simulink model "main"  (R2023a)
settings: Solver=VariableStepAuto  StartTime=0.0  StopTime=20.0  RelTol=1e-3
values from neighbouring files (symbols this model uses):
  K_cor = -321.168335055129    (= -321.168335055)    [init_constants.m]
  K_d = -25.0617020806048    (= -25.0617020806)    [init_constants.m]
  K_i = -1.34615707043330    (= -1.34615707043)    [init_constants.m]
  K_m = 1    [init_constants.m]
  K_p = 29.6159033557395    (= 29.6159033557)    [init_constants.m]
libraries: checkpacklib x1
settings Model: Creator=agalimov  LastModifiedBy=agalimov

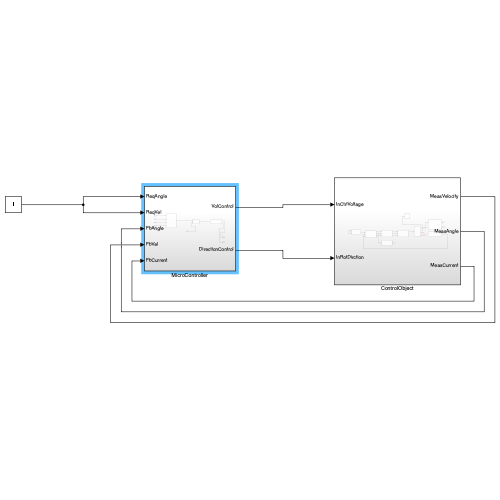
[thumbnail: Simulink's stored preview of the top-level diagram]
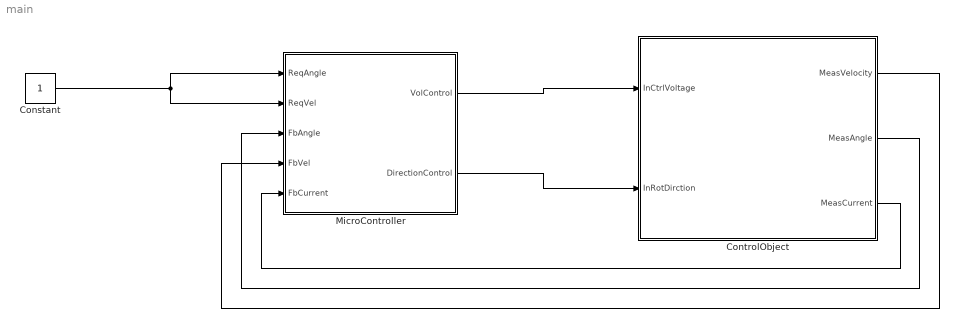
== system main ==
  Constant : Constant
  ControlObject : Subsystem
  MicroController : Subsystem
  wires:
  MicroController/1(VolControl) -> ControlObject/1(InCtrlVoltage)
  ControlObject/3(MeasCurrent) -> MicroController/5(FbCurrent)
  ControlObject/2(MeasAngle) -> MicroController/3(FbAngle)
  ControlObject/1(MeasVelocity) -> MicroController/4(FbVel)
  Constant/1 -> MicroController/2(ReqVel), MicroController/1(ReqAngle)
  MicroController/2(DirectionControl) -> ControlObject/2(InRotDirction)

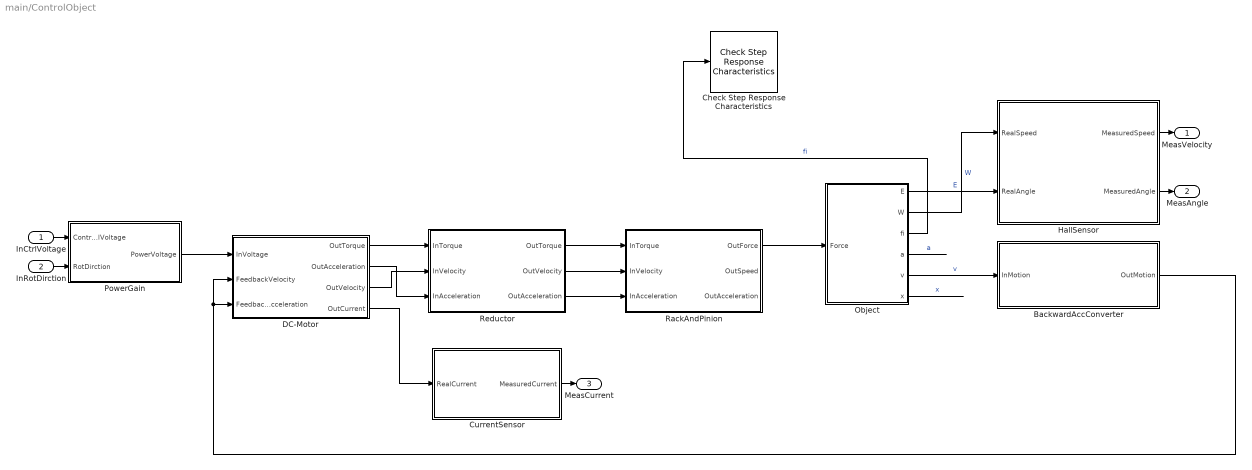
== system main/ControlObject ==
  InCtrlVoltage : Inport
  InRotDirction : Inport  Port=2
  BackwardAccConverter : Subsystem
  Check Step Response Characteristics : checkpacklib/Check Step Response  Characteristics  InstantiateOnLoad=on  enabled=on  stopWhenAssertionFail=off  export=off  ViewDlgPos=[]  OpenViewOnLoad=off  LaunchViewOnOpen=off  TimeUnits=seconds  EnableStepResponseBound=on  InitialValue=0  FinalValue=1  StepTime=0  RiseTime=5  PercentRise=80  SettlingTime=7  PercentSettling=1  PercentOvershoot=10  PercentUndershoot=1
      settings: LibrarySourceBlock=|
      | sdolib/Model Verification/Check Step Response
      | Characteristics
  CurrentSensor : Subsystem
  DC-Motor : Subsystem  mask{R=10, L=0.000350, kw=10, km=0.016, J_motor=0.0000005, vis_friction_coef_motor=0.5}
      mask prompts: R "Активное сопротивление якоря, Ом"; L "Индуктивность якоря, Гн"; kw "Коэф. скорости двигателя, об/сек"; km "Коэф. момента двигателя, Н*м/А"; J_motor "Момент инерции, кг*м^2"; vis_friction_coef_motor "Коэф. вязкого трения двигателя"
  HallSensor : Subsystem
  Object : Subsystem
  PowerGain : Subsystem  mask{Gain_=8, Saturation_=24}
      mask prompts: Gain_ "Gain"; Saturation_ "Saturation"
  RackAndPinion : Subsystem  mask{vis_friction_coef_gear=0.5, i_rack=20000, J_rack=0.000001, m=0.3}
      mask prompts: vis_friction_coef_gear "Коэф. вязкого трения"; i_rack "Передаточное отношение, рад/м"; J_rack "Момент инерции"; m "Масса маятника, кг"
  Reductor : Subsystem  mask{i_gear=100, J_gear=0.000024, vis_friction_coef_gear=0.5}
      mask prompts: i_gear "Передаточное отношение"; J_gear "Момент инерции, кг*м^2"; vis_friction_coef_gear "Коэф. вязкого трения редуктора"
  MeasVelocity : Outport
  MeasAngle : Outport  Port=2
  MeasCurrent : Outport  Port=3
  wires:
  Reductor/3(OutAcceleration) -> RackAndPinion/3(InAcceleration)
  Reductor/2(OutVelocity) -> RackAndPinion/2(InVelocity)
  HallSensor/2(MeasuredAngle) -> MeasAngle/1
  DC-Motor/4(OutCurrent) -> CurrentSensor/1(RealCurrent)
  Reductor/1(OutTorque) -> RackAndPinion/1(InTorque)
  DC-Motor/3(OutVelocity) -> Reductor/2(InVelocity)
  DC-Motor/1(OutTorque) -> Reductor/1(InTorque)
  BackwardAccConverter/1(OutMotion) -> DC-Motor/3(FeedbackAcceleration), DC-Motor/2(FeedbackVelocity)
  HallSensor/1(MeasuredSpeed) -> MeasVelocity/1
  DC-Motor/2(OutAcceleration) -> Reductor/3(InAcceleration)
  PowerGain/1(PowerVoltage) -> DC-Motor/1(InVoltage)
  CurrentSensor/1(MeasuredCurrent) -> MeasCurrent/1
  InCtrlVoltage/1 -> PowerGain/1(ControlVoltage)
  InRotDirction/1 -> PowerGain/2(RotDirction)
  Object/5(v) -> BackwardAccConverter/1(InMotion)  "v"
  Object/2(W) -> HallSensor/1(RealSpeed)  "W"
  Object/1(E) -> HallSensor/2(RealAngle)  "E"
  RackAndPinion/1(OutForce) -> Object/1(Force)
  Object/3(fi) -> Check Step Response Characteristics/1  "fi"
  Object/4(a) -> ?  "a"
  Object/6(x) -> ?  "x"

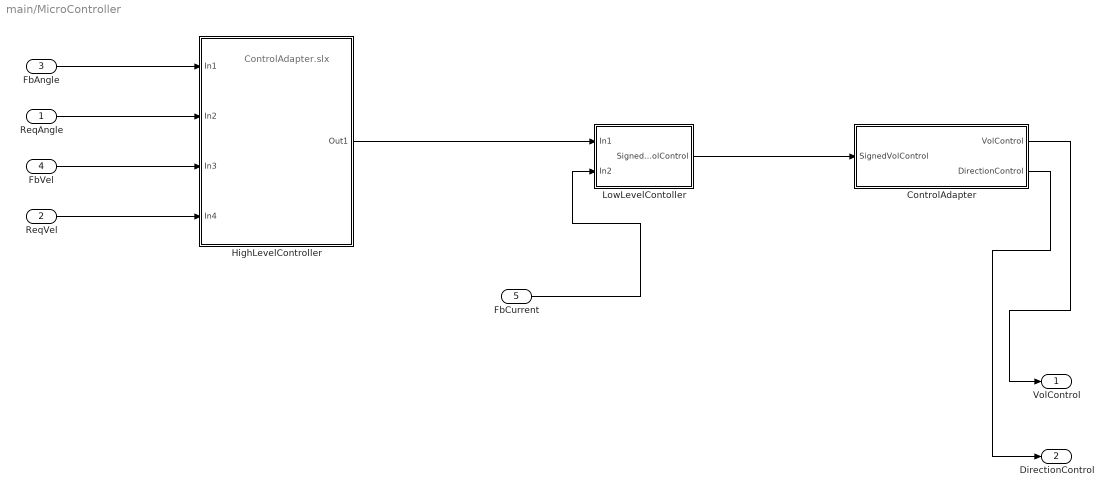
== system main/MicroController ==
  note: ControlAdapter.slx
  ReqAngle : Inport
  ReqVel : Inport  Port=2
  FbAngle : Inport  Port=3
  FbVel : Inport  Port=4
  FbCurrent : Inport  Port=5
  ControlAdapter : Subsystem
  HighLevelController : Subsystem
  LowLevelContoller : Subsystem
  VolControl : Outport
  DirectionControl : Outport  Port=2  OutDataTypeStr=boolean
  wires:
  FbAngle/1 -> HighLevelController/1(In1)
  ReqAngle/1 -> HighLevelController/2(In2)
  FbVel/1 -> HighLevelController/3(In3)
  ReqVel/1 -> HighLevelController/4(In4)
  HighLevelController/1(Out1) -> LowLevelContoller/1(In1)
  FbCurrent/1 -> LowLevelContoller/2(In2)
  LowLevelContoller/1(SignedVolControl) -> ControlAdapter/1(SignedVolControl)
  ControlAdapter/1(VolControl) -> VolControl/1
  ControlAdapter/2(DirectionControl) -> DirectionControl/1

== system main/ControlObject/BackwardAccConverter ==
  InMotion : Inport
  Gain2 : Gain  Gain=1 /(100*20000)
  OutMotion : Outport
  wires:
  InMotion/1 -> Gain2/1
  Gain2/1 -> OutMotion/1

== system main/ControlObject/CurrentSensor ==
  RealCurrent : Inport
  Gain : Gain  Gain=0.001
  MeasuredCurrent : Outport
  wires:
  Gain/1 -> MeasuredCurrent/1
  RealCurrent/1 -> Gain/1

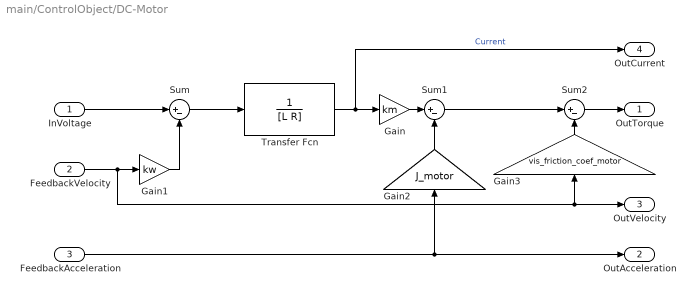
== system main/ControlObject/DC-Motor ==
  InVoltage : Inport
  FeedbackVelocity : Inport  Port=2
  FeedbackAcceleration : Inport  Port=3
  Gain : Gain  Gain=km
  Gain1 : Gain  Gain=kw
  Gain2 : Gain  Gain=J_motor
  Gain3 : Gain  Gain=vis_friction_coef_motor
  Sum : Sum  Inputs=|+-
  Sum1 : Sum  Inputs=|+-
  Sum2 : Sum  Inputs=|+-
  Transfer Fcn : TransferFcn  Denominator=[L R]
  OutTorque : Outport
  OutAcceleration : Outport  Port=2
  OutVelocity : Outport  Port=3
  OutCurrent : Outport  Port=4
  wires:
  InVoltage/1 -> Sum/1
  Sum/1 -> Transfer Fcn/1
  Transfer Fcn/1 -> OutCurrent/1, Gain/1  "Current"
  FeedbackVelocity/1 -> OutVelocity/1, Gain3/1, Gain1/1
  Gain1/1 -> Sum/2
  FeedbackAcceleration/1 -> OutAcceleration/1, Gain2/1
  Gain/1 -> Sum1/1
  Gain2/1 -> Sum1/2
  Sum1/1 -> Sum2/1
  Sum2/1 -> OutTorque/1
  Gain3/1 -> Sum2/2

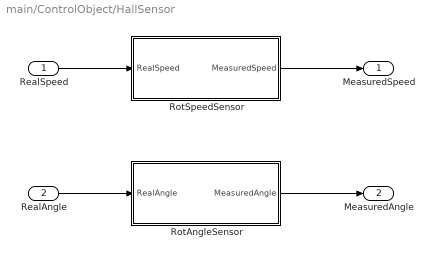
== system main/ControlObject/HallSensor ==
  RealSpeed : Inport
  RealAngle : Inport  Port=2
  RotAngleSensor : Subsystem
  RotSpeedSensor : Subsystem
  MeasuredSpeed : Outport
  MeasuredAngle : Outport  Port=2
  wires:
  RotSpeedSensor/1(MeasuredSpeed) -> MeasuredSpeed/1
  RealAngle/1 -> RotAngleSensor/1(RealAngle)
  RealSpeed/1 -> RotSpeedSensor/1(RealSpeed)
  RotAngleSensor/1(MeasuredAngle) -> MeasuredAngle/1

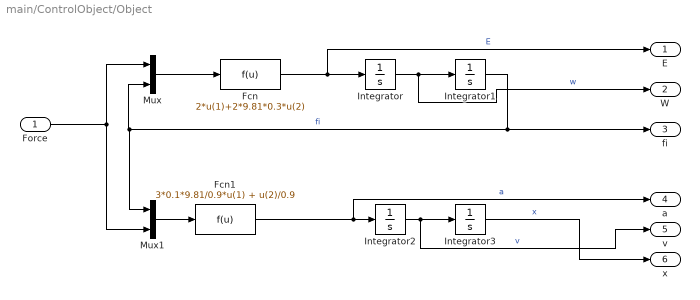
== system main/ControlObject/Object ==
  Force : Inport
  Fcn : Fcn  Expr=2*u(1)+2*9.81*0.3*u(2)
  Fcn1 : Fcn  Expr=3*0.1*9.81/0.9*u(1) + u(2)/0.9
  Integrator : Integrator
  Integrator1 : Integrator  InitialCondition=0.0873
  Integrator2 : Integrator
  Integrator3 : Integrator
  Mux : Mux  Inputs=2
  Mux1 : Mux  Inputs=2
  E : Outport
  W : Outport  Port=2
  fi : Outport  Port=3
  a : Outport  Port=4
  v : Outport  Port=5
  x : Outport  Port=6
  wires:
  Fcn1/1 -> a/1, Integrator2/1  "a"
  Integrator3/1 -> x/1  "x"
  Integrator2/1 -> v/1, Integrator3/1  "v"
  Fcn/1 -> E/1, Integrator/1  "E"
  Force/1 -> Mux1/2, Mux/1
  Integrator/1 -> W/1, Integrator1/1  "w"
  Integrator1/1 -> Mux1/1, Mux/2, fi/1  "fi"
  Mux1/1 -> Fcn1/1
  Mux/1 -> Fcn/1

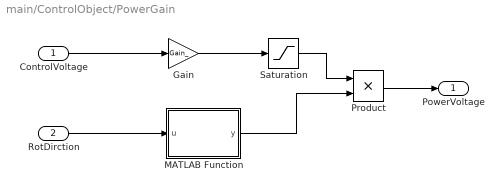
== system main/ControlObject/PowerGain ==
  ControlVoltage : Inport
  RotDirction : Inport  Port=2  OutDataTypeStr=boolean
  Gain : Gain  Gain=Gain_
  MATLAB Function : MATLAB Function  TreatAsAtomicUnit=on
  Product : Product
  Saturation : Saturate  UpperLimit=Saturation_  LowerLimit=0
  PowerVoltage : Outport
  wires:
  Gain/1 -> Saturation/1
  ControlVoltage/1 -> Gain/1
  RotDirction/1 -> MATLAB Function/1(u)
  MATLAB Function/1(y) -> Product/2
  Saturation/1 -> Product/1
  Product/1 -> PowerVoltage/1

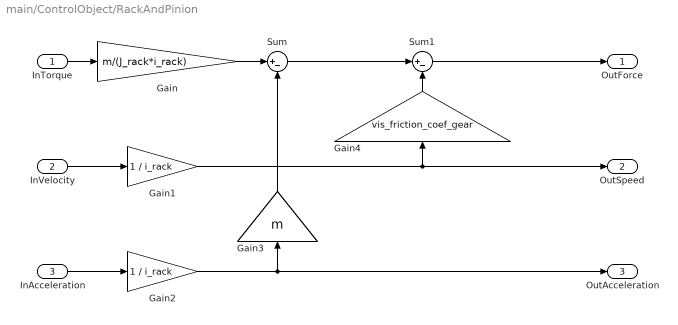
== system main/ControlObject/RackAndPinion ==
  InTorque : Inport
  InVelocity : Inport  Port=2
  InAcceleration : Inport  Port=3
  Gain : Gain  Gain=m/(J_rack*i_rack)
  Gain1 : Gain  Gain=1 / i_rack
  Gain2 : Gain  Gain=1 / i_rack
  Gain3 : Gain  Gain=m
  Gain4 : Gain  Gain=vis_friction_coef_gear
  Sum : Sum  Inputs=|+-
  Sum1 : Sum  Inputs=|+-
  OutForce : Outport
  OutSpeed : Outport  Port=2
  OutAcceleration : Outport  Port=3
  wires:
  InTorque/1 -> Gain/1
  InVelocity/1 -> Gain1/1
  InAcceleration/1 -> Gain2/1
  Gain2/1 -> Gain3/1, OutAcceleration/1
  Gain1/1 -> Gain4/1, OutSpeed/1
  Gain/1 -> Sum/1
  Sum/1 -> Sum1/1
  Sum1/1 -> OutForce/1
  Gain3/1 -> Sum/2
  Gain4/1 -> Sum1/2

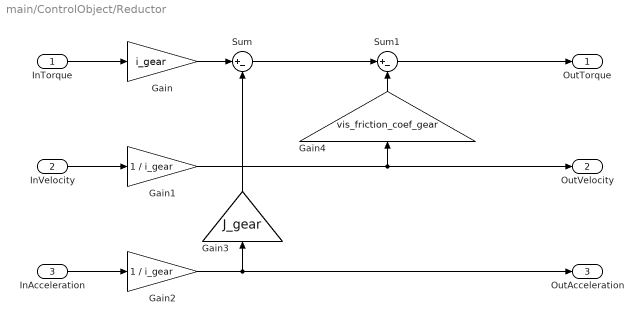
== system main/ControlObject/Reductor ==
  InTorque : Inport
  InVelocity : Inport  Port=2
  InAcceleration : Inport  Port=3
  Gain : Gain  Gain=i_gear
  Gain1 : Gain  Gain=1 / i_gear
  Gain2 : Gain  Gain=1 / i_gear
  Gain3 : Gain  Gain=J_gear
  Gain4 : Gain  Gain=vis_friction_coef_gear
  Sum : Sum  Inputs=|+-
  Sum1 : Sum  Inputs=|+-
  OutTorque : Outport
  OutVelocity : Outport  Port=2
  OutAcceleration : Outport  Port=3
  wires:
  InTorque/1 -> Gain/1
  InVelocity/1 -> Gain1/1
  InAcceleration/1 -> Gain2/1
  Gain2/1 -> Gain3/1, OutAcceleration/1
  Gain1/1 -> Gain4/1, OutVelocity/1
  Gain/1 -> Sum/1
  Sum/1 -> Sum1/1
  Sum1/1 -> OutTorque/1
  Gain3/1 -> Sum/2
  Gain4/1 -> Sum1/2

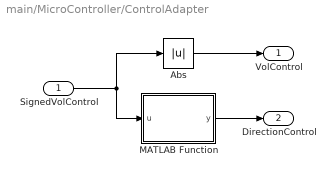
== system main/MicroController/ControlAdapter ==
  SignedVolControl : Inport
  Abs : Abs  SaturateOnIntegerOverflow=off
  MATLAB Function : MATLAB Function  TreatAsAtomicUnit=on
  VolControl : Outport
  DirectionControl : Outport  Port=2  OutDataTypeStr=boolean
  wires:
  Abs/1 -> VolControl/1
  SignedVolControl/1 -> MATLAB Function/1(u), Abs/1
  MATLAB Function/1(y) -> DirectionControl/1

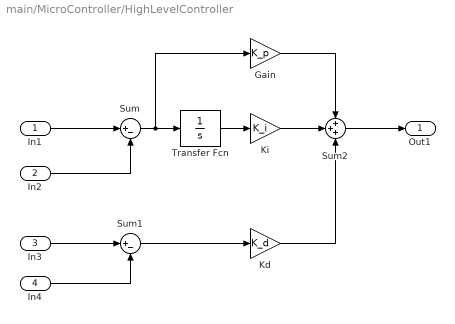
== system main/MicroController/HighLevelController ==
  In1 : Inport
  In2 : Inport  Port=2
  In3 : Inport  Port=3
  In4 : Inport  Port=4
  Gain : Gain  Gain=K_p
  Kd : Gain  Gain=K_d
  Ki : Gain  Gain=K_i
  Sum : Sum  Inputs=|+-
  Sum1 : Sum  Inputs=|+-
  Sum2 : Sum  Inputs=+++
  Transfer Fcn : TransferFcn  Denominator=[1 0]
  Out1 : Outport
  wires:
  Ki/1 -> Sum2/2
  Sum/1 -> Gain/1, Transfer Fcn/1
  Kd/1 -> Sum2/3
  Gain/1 -> Sum2/1
  In4/1 -> Sum1/2
  In2/1 -> Sum/2
  Sum1/1 -> Kd/1
  Transfer Fcn/1 -> Ki/1
  Sum2/1 -> Out1/1
  In3/1 -> Sum1/1
  In1/1 -> Sum/1

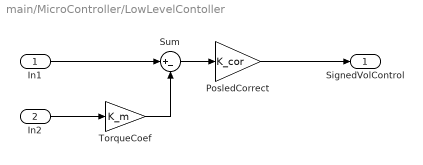
== system main/MicroController/LowLevelContoller ==
  In1 : Inport
  In2 : Inport  Port=2
  PosledCorrect : Gain  Gain=K_cor
  Sum : Sum  Inputs=|+-
  TorqueCoef : Gain  Gain=K_m
  SignedVolControl : Outport
  wires:
  In1/1 -> Sum/1
  Sum/1 -> PosledCorrect/1
  In2/1 -> TorqueCoef/1
  PosledCorrect/1 -> SignedVolControl/1
  TorqueCoef/1 -> Sum/2

== system main/ControlObject/HallSensor/RotAngleSensor ==
  RealAngle : Inport
  Gain1 : Gain  Gain=2
  MeasuredAngle : Outport
  wires:
  Gain1/1 -> MeasuredAngle/1
  RealAngle/1 -> Gain1/1

== system main/ControlObject/HallSensor/RotSpeedSensor ==
  RealSpeed : Inport
  Gain : Gain  Gain=0.2
  MeasuredSpeed : Outport
  wires:
  RealSpeed/1 -> Gain/1
  Gain/1 -> MeasuredSpeed/1

== matlab function main/ControlObject/PowerGain/MATLAB Function ==
  data: u input; y output
function y = fcn(u)
if u == true
    y = 1;
else
    y = -1;
end

== matlab function main/MicroController/ControlAdapter/MATLAB Function ==
  data: u input; y output
function y = fcn(u)
if u>0
    y=true;
else
    y=false;
end
